simulink model "sideslip_tune"  (R2016a)
settings: Solver=VariableStepAuto  StartTime=0.0  StopTime=10.0  RelTol=1e-3
values from neighbouring files (symbols this model uses):
  a_beta1 = 0.4785    [tune_sideslip.m]
  a_beta2 = -2.9051    [tune_sideslip.m]
  beta_ki = wn_beta^2 / a_beta2    (= -0.101998555518)    [tune_sideslip.m]
  beta_kp = -delta_r_max / vr_max    (= -0.116355283466)    [tune_sideslip.m]
settings Model: Creator=andreanv  LastModifiedBy=andreanv

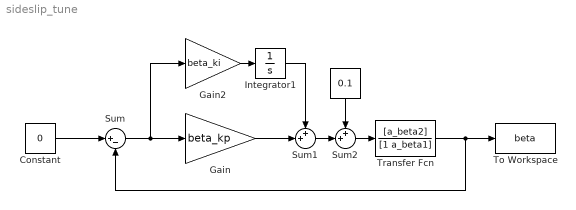
== system sideslip_tune ==
  " " : Constant  Value=0.1
  Constant : Constant  Value=0
  Gain : Gain  Gain=beta_kp
  Gain2 : Gain  Gain=beta_ki
  Integrator1 : Integrator
  Sum : Sum  Inputs=|+-
  Sum1 : Sum  Inputs=++|
  Sum2 : Sum  Inputs=++|
  To Workspace : ToWorkspace  VariableName=beta  SaveFormat=Timeseries  SampleTime=-1
  Transfer Fcn : TransferFcn  Numerator=[a_beta2]  Denominator=[1 a_beta1]
  wires:
  Constant/1 -> Sum/1
  Sum/1 -> Gain2/1, Gain/1
  Sum1/1 -> Sum2/2
  Sum2/1 -> Transfer Fcn/1
  " "/1 -> Sum2/1
  Gain2/1 -> Integrator1/1
  Integrator1/1 -> Sum1/1
  Gain/1 -> Sum1/2
  Transfer Fcn/1 -> Sum/2, To Workspace/1
